simulink model "clase_04_may"  (R2021a)
settings: Solver=VariableStepAuto  StartTime=0.0  StopTime=10.0  RelTol=1e-3
settings Model: Creator=pierr  LastModifiedBy=pierr

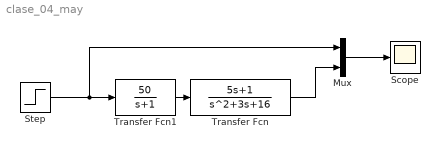
== system clase_04_may ==
  Mux : Mux  Inputs=2
  Scope : Scope
  Step : Step  SampleTime=0
  Transfer Fcn : TransferFcn  Numerator=[5 1]  Denominator=[1 3 16]
  Transfer Fcn1 : TransferFcn  Numerator=[50]  Denominator=[1 1]
  wires:
  Transfer Fcn1/1 -> Transfer Fcn/1
  Transfer Fcn/1 -> Mux/2
  Step/1 -> Mux/1, Transfer Fcn1/1
  Mux/1 -> Scope/1
